simulink model "EQM"  (Simulink 7.8)
settings: Solver=FixedStepDiscrete  SolverMode=SingleTasking  StartTime=0.0  StopTime=t_end  FixedStep=dt_control  RelTol=1e-3
values from neighbouring files (symbols this model uses):
  dt_sim = 0.005    [Init.m]
  J = diag([0.25*m*(D/2)^2 0.25*m*(D/2)^2 0.5*m*(D/2)^2])    [Init.m]
  m = 1    [Init.m]
libraries: simulink x1
settings Model: Creator=ft14sl  LastModifiedBy=ft14sl
settings DataIOCC: LimitDataPoints=off  SaveOutput=off  SignalLogging=off  DSMLogging=off  SaveTime=off
settings DebuggingCC: ConsistencyChecking=error  SignalInfNanChecking=error  SignalRangeChecking=error  AlgebraicLoopMsg=error  ArtificialAlgebraicLoopMsg=error  SaveWithDisabledLinksMsg=error  SaveWithParameterizedLinksMsg=error  UnderspecifiedInitializationDetection=Simplified  MergeDetectMultiDrivingBlocksExec=error  BlockPriorityViolationMsg=error  MinStepSizeMsg=error  TimeAdjustmentMsg=warning  SolverPrmCheckMsg=error  InheritedTsInSrcMsg=error  DiscreteInheritContinuousMsg=error  SingleTaskRateTransMsg=error  TasksWithSamePriorityMsg=error  SigSpecEnsureSampleTimeMsg=error  CheckMatrixSingularityMsg=error  IntegerOverflowMsg=error  ParameterUnderflowMsg=error  ParameterPrecisionLossMsg=error  ParameterTunabilityLossMsg=error  FixptConstUnderflowMsg=error  FixptConstOverflowMsg=error  FixptConstPrecisionLossMsg=error  UnderSpecifiedDataTypeMsg=error  UnnecessaryDatatypeConvMsg=warning  VectorMatrixConversionMsg=error  SignalLabelMismatchMsg=error  UnconnectedInputMsg=error  UnconnectedOutputMsg=error  UnconnectedLineMsg=error  SFcnCompatibilityMsg=error  UniqueDataStoreMsg=error  BusObjectLabelMismatch=error  RootOutportRequireBusObject=error  ModelReferenceIOMsg=error  ModelReferenceVersionMismatchMessage=error  ModelReferenceIOMismatchMessage=error  ModelReferenceCSMismatchMessage=error  UnknownTsInhSupMsg=error  ModelReferenceDataLoggingMessage=error  SimStateInterfaceChecksumMismatchMsg=error  StrictBusMsg=ErrorOnBusTreatedAsVector  NonBusSignalsTreatedAsBus=error  SFUnusedDataAndEventsDiag=error  SFUnexpectedBacktrackingDiag=error  SFInvalidInputDataAccessInChartInitDiag=error  SFNoUnconditionalDefaultTransitionDiag=error  SFTransitionOutsideNaturalParentDiag=error  SFUnconditionalTransitionShadowingDiag=error

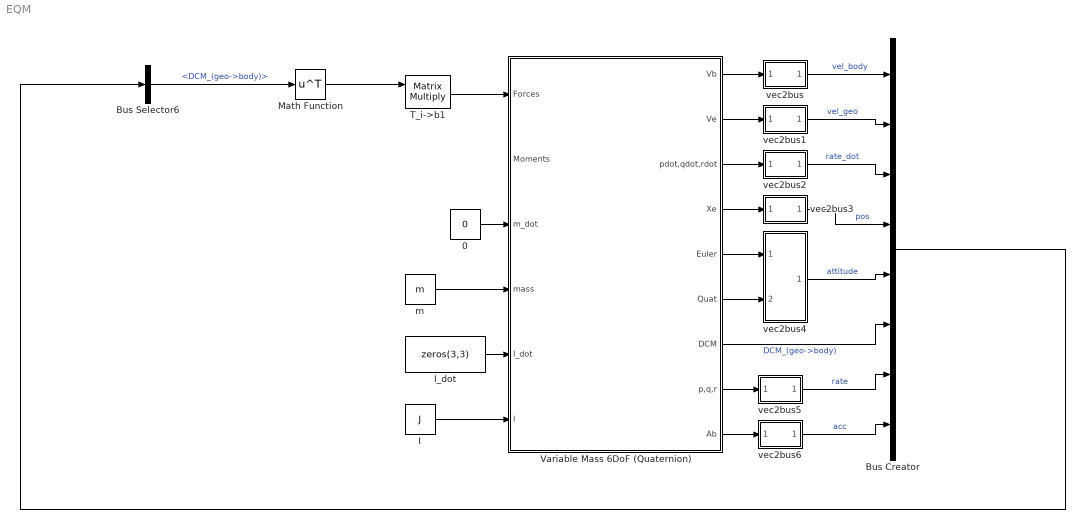
== system EQM ==
  0 : Constant  Value=0
  Bus Creator : BusCreator  Inputs=8
  Bus Selector6 : BusSelector  OutputSignals=DCM_(geo->body)
  I : Constant  Value=J
  I_dot : Constant  Value=zeros(3,3)
  Math Function : Math  Operator=transpose  SaturateOnIntegerOverflow=on
  T_i->b1 : Product  Multiplication=Matrix(*)  SaturateOnIntegerOverflow=on  OutDataTypeStr=Inherit: Same as first input
  Variable Mass 6DoF (Quaternion) : Subsystem  mask{xme_0=[0 0 0], Vm_0=[0 0 0], eul_0=[0 0 0], pm_0=[0 0 0], dt_sim=dt_sim}
      mask prompts: xme_0 "Inertial position in inertial axes [Xe, Ye Ze]"; Vm_0 "Inertial velocity in body axes [u, v, w]"; eul_0 "Inertial Euler orientation [roll, pitch, yaw]"; pm_0 "Inertial body rotation rates[p, q, r]"; dt_sim "Sample Time for quaternion integration"
      mask help:
      | Variable Mass 6DoF (Quaternion)
      | (rebuild from MATLAB AeroSpace Blockset)
      mask Help:
      | Inputs and Outputs
      | 
      | The first input to the block is a vector containing the three applied forces.
      | The second input is a vector containing the three applied moments.
      | The third input is a scalar containing the rate of change of mass.
      | The fourth input is a scalar containing the mass
      | The fifth input is a 3-by-3 matrix for the rate of change of inertia tensor matrix.
      | The sixth input is a 3-by-3 matrix for the inertia tensor matrix.
      | 
      | The first output is a three-element vector containing the velocity in the Earth-fixed reference frame.
      | The second output is a three-element vector containing the position in the Earth-fixed reference frame.
      | The third output is a three-element vector containing the Euler rotation angles [roll, pitch, yaw], in radians.
      | The fourth output is a 3-by-3 matrix for the coordinate transformation from Earth-fixed axes to body-fixed axes.
      | The fifth output is a three-element vector containing the velocity in the body-fixed frame.
      | The sixth output is a three-element vector containing the angular rates in body-fixed axes, in radians per second.
      | The seventh output is a three-element vector containing the angular accelerations in body-fixed axes, in radians per second. The eighth output is a three-element vector containing the accelerations in body-fixed axes.
      mask Display:
      | port_label('input',1,'F_xyz (N)')
      | port_label('input',2,'M_xyz (Nm)')
      | port_label('input',3,'dm/dt (kg/s)')
      | port_label('input',4,'m (kg)')
      | port_label('input',5,'dI/dt (kgm^2/s)')
      | port_label('input',6,'I (kgm^2)')
      | port_label('output',1,'Vb (m/s)')
      | port_label('output',2,'Ve (m/s)')
      | port_label('output',3,'pqrdot')
      | port_label('output',4,'Xe')
      | port_label('output',5,'phi theta psi (rad)')
      | port_label('output',6,'quaternions')
      | port_label('output',7,'DCM')
      | port_label('output',8,'pqr')
      | port_label('output',9,'Ab (m/s^2)')
  m : Constant  Value=m
  vec2bus : Subsystem
  vec2bus1 : Subsystem
  vec2bus2 : Subsystem
  vec2bus3 : Subsystem
  vec2bus4 : Subsystem
  vec2bus5 : Subsystem
  vec2bus6 : Subsystem
  wires:
  T_i->b1/1 -> Variable Mass 6DoF (Quaternion)/1(Forces)
  vec2bus6/1(bus) -> Bus Creator/8  "acc"
  vec2bus5/1(bus) -> Bus Creator/7  "rate"
  Variable Mass 6DoF (Quaternion)/7(DCM) -> Bus Creator/6  "DCM_(geo->body)"
  vec2bus4/1(bus) -> Bus Creator/5  "attitude"
  vec2bus3/1(bus) -> Bus Creator/4  "pos"
  vec2bus2/1(bus) -> Bus Creator/3  "rate_dot"
  vec2bus1/1(bus) -> Bus Creator/2  "vel_geo"
  vec2bus/1(bus) -> Bus Creator/1  "vel_body"
  Variable Mass 6DoF (Quaternion)/6(Quat) -> vec2bus4/2(quat)
  Variable Mass 6DoF (Quaternion)/9(Ab) -> vec2bus6/1(vec)
  Variable Mass 6DoF (Quaternion)/8(p,q,r) -> vec2bus5/1(vec)
  Variable Mass 6DoF (Quaternion)/5(Euler) -> vec2bus4/1(euler)
  Variable Mass 6DoF (Quaternion)/4(Xe) -> vec2bus3/1(vec)
  Variable Mass 6DoF (Quaternion)/3(pdot,qdot,rdot) -> vec2bus2/1(vec)
  Variable Mass 6DoF (Quaternion)/2(Ve) -> vec2bus1/1(vec)
  Variable Mass 6DoF (Quaternion)/1(Vb) -> vec2bus/1(vec)
  I/1 -> Variable Mass 6DoF (Quaternion)/6(I)
  I_dot/1 -> Variable Mass 6DoF (Quaternion)/5(I_dot)
  m/1 -> Variable Mass 6DoF (Quaternion)/4(mass)
  0/1 -> Variable Mass 6DoF (Quaternion)/3(m_dot)
  Math Function/1 -> T_i->b1/1
  Bus Selector6/1 -> Math Function/1  "<DCM_(geo->body)>"
  Bus Creator/1 -> Bus Selector6/1

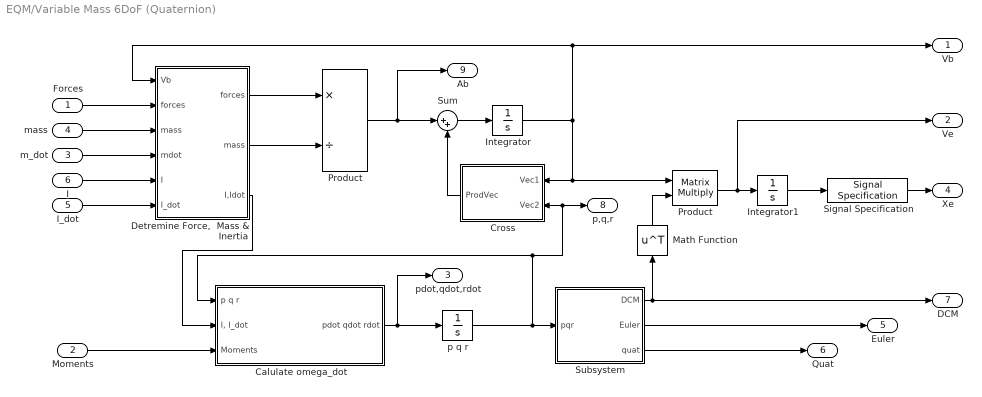
== system EQM/Variable Mass 6DoF (Quaternion) ==
  Forces : Inport
  Moments : Inport  Port=2
  m_dot : Inport  Port=3
  mass : Inport  Port=4
  I_dot : Inport  Port=5
  I : Inport  Port=6
  Calulate omega_dot : Subsystem
  Cross : Subsystem
  "Detremine Force,  Mass & Inertia" : Subsystem
  Integrator : Integrator  InitialCondition=Vm_0
  Integrator1 : Integrator  InitialCondition=xme_0
  Math Function : Math  Operator=transpose  SaturateOnIntegerOverflow=on
  Product : Product  Inputs=*/  SaturateOnIntegerOverflow=on  OutDataTypeStr=Inherit: Same as first input
  "Product " : Product  Multiplication=Matrix(*)  SaturateOnIntegerOverflow=on  OutDataTypeStr=Inherit: Same as first input
  Signal Specification : SignalSpecification  OutDataTypeStr=double
  Subsystem : Subsystem
  Sum : Sum  Inputs=|++  SaturateOnIntegerOverflow=on
  p q r : Integrator
  Vb : Outport
  Ve : Outport  Port=2
  pdot,qdot,rdot : Outport  Port=3
  Xe : Outport  Port=4
  Euler : Outport  Port=5
  Quat : Outport  Port=6
  DCM : Outport  Port=7
  p,q,r : Outport  Port=8
  Ab : Outport  Port=9
  wires:
  Subsystem/2(Euler) -> Euler/1
  Integrator1/1 -> Signal Specification/1
  "Product "/1 -> Ve/1, Integrator1/1
  "Detremine Force,  Mass & Inertia"/3(I,Idot) -> Calulate omega_dot/2("I, I_dot")
  Moments/1 -> Calulate omega_dot/3(Moments)
  Calulate omega_dot/1(pdot qdot rdot) -> pdot,qdot,rdot/1, p q r/1
  p q r/1 -> Calulate omega_dot/1(p q r), Cross/2(Vec2), p,q,r/1, Subsystem/1(pqr)
  Subsystem/1(DCM) -> DCM/1, Math Function/1
  Math Function/1 -> "Product "/2
  Cross/1(ProdVec) -> Sum/2
  Sum/1 -> Integrator/1
  Integrator/1 -> Vb/1, "Detremine Force,  Mass & Inertia"/1(Vb), "Product "/1, Cross/1(Vec1)
  Product/1 -> Sum/1, Ab/1
  "Detremine Force,  Mass & Inertia"/2("mass ") -> Product/2
  "Detremine Force,  Mass & Inertia"/1("forces ") -> Product/1
  I_dot/1 -> "Detremine Force,  Mass & Inertia"/6(I_dot)
  I/1 -> "Detremine Force,  Mass & Inertia"/5(I)
  m_dot/1 -> "Detremine Force,  Mass & Inertia"/4(mdot)
  mass/1 -> "Detremine Force,  Mass & Inertia"/3(mass)
  Forces/1 -> "Detremine Force,  Mass & Inertia"/2(forces)
  Subsystem/3(quat) -> Quat/1
  Signal Specification/1 -> Xe/1

== system EQM/vec2bus ==
  vec : Inport
  Bus Creator : BusCreator  Inputs=3
  Demux : Demux  Outputs=3
  bus : Outport
  wires:
  Demux/1 -> Bus Creator/1  "ub"
  Demux/2 -> Bus Creator/2  "vb"
  Demux/3 -> Bus Creator/3  "wb"
  Bus Creator/1 -> bus/1
  vec/1 -> Demux/1

== system EQM/vec2bus1 ==
  vec : Inport
  Bus Creator : BusCreator  Inputs=3
  Demux : Demux  Outputs=3
  bus : Outport
  wires:
  vec/1 -> Demux/1
  Bus Creator/1 -> bus/1
  Demux/3 -> Bus Creator/3  "wg"
  Demux/2 -> Bus Creator/2  "vg"
  Demux/1 -> Bus Creator/1  "ug"

== system EQM/vec2bus2 ==
  vec : Inport
  Bus Creator : BusCreator  Inputs=3
  Demux : Demux  Outputs=3
  bus : Outport
  wires:
  Demux/1 -> Bus Creator/1  "pdot"
  Demux/2 -> Bus Creator/2  "qdot"
  Demux/3 -> Bus Creator/3  "rdot"
  Bus Creator/1 -> bus/1
  vec/1 -> Demux/1

== system EQM/vec2bus3 ==
  vec : Inport
  Bus Creator : BusCreator  Inputs=3
  Demux : Demux  Outputs=3
  bus : Outport
  wires:
  vec/1 -> Demux/1
  Bus Creator/1 -> bus/1
  Demux/3 -> Bus Creator/3  "z"
  Demux/2 -> Bus Creator/2  "y"
  Demux/1 -> Bus Creator/1  "x"

== system EQM/vec2bus4 ==
  euler : Inport
  quat : Inport  Port=2
  Bus Creator : BusCreator  Inputs=7
  Demux : Demux  Outputs=3
  Demux1 : Demux
  bus : Outport
  wires:
  Demux/1 -> Bus Creator/1  "phi"
  Demux/2 -> Bus Creator/2  "theta"
  Demux/3 -> Bus Creator/3  "psi"
  Demux1/1 -> Bus Creator/4
  Demux1/2 -> Bus Creator/5
  Demux1/3 -> Bus Creator/6
  Demux1/4 -> Bus Creator/7
  euler/1 -> Demux/1
  Bus Creator/1 -> bus/1
  quat/1 -> Demux1/1

== system EQM/vec2bus5 ==
  vec : Inport
  Bus Creator : BusCreator  Inputs=3
  Demux : Demux  Outputs=3
  bus : Outport
  wires:
  vec/1 -> Demux/1
  Bus Creator/1 -> bus/1
  Demux/3 -> Bus Creator/3  "r"
  Demux/2 -> Bus Creator/2  "q"
  Demux/1 -> Bus Creator/1  "p"

== system EQM/vec2bus6 ==
  vec : Inport
  Bus Creator : BusCreator  Inputs=3
  Demux : Demux  Outputs=3
  bus : Outport
  wires:
  Demux/1 -> Bus Creator/1  "ax"
  Demux/2 -> Bus Creator/2  "ay"
  Demux/3 -> Bus Creator/3  "az"
  Bus Creator/1 -> bus/1
  vec/1 -> Demux/1

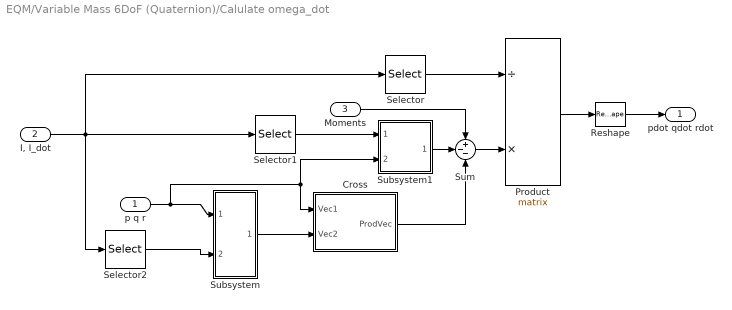
== system EQM/Variable Mass 6DoF (Quaternion)/Calulate omega_dot ==
  p q r : Inport
  "I, I_dot" : Inport  Port=2
  Moments : Inport  Port=3
  Cross : Subsystem
  Product : Product  Inputs=/*  Multiplication=Matrix(*)  SaturateOnIntegerOverflow=on  OutDataTypeStr=Inherit: Same as first input
  Reshape : Reshape
  Selector : Selector  NumberOfDimensions=2  InputPortWidth=3  IndexOptions=Index vector (dialog),Select all  Indices=1:3,-1  OutputSizes=1
  Selector1 : Selector  NumberOfDimensions=2  InputPortWidth=3  IndexOptions=Index vector (dialog),Select all  Indices=4:6,-1  OutputSizes=1
  Selector2 : Selector  NumberOfDimensions=2  InputPortWidth=3  IndexOptions=Index vector (dialog),Select all  Indices=1:3,-1  OutputSizes=1
  Subsystem : Subsystem
  Subsystem1 : Subsystem
  Sum : Sum  Inputs=+--  SaturateOnIntegerOverflow=on
  pdot qdot rdot : Outport
  wires:
  Cross/1(ProdVec) -> Sum/3
  Product/1 -> Reshape/1
  Subsystem/1(I*w) -> Cross/2(Vec2)
  Selector2/1 -> Subsystem/2(Inertia)
  p q r/1 -> Subsystem1/2(p q r), Cross/1(Vec1), Subsystem/1(p q r)
  Moments/1 -> Sum/1
  Reshape/1 -> pdot qdot rdot/1
  Sum/1 -> Product/2
  Subsystem1/1(Id*w) -> Sum/2
  Selector1/1 -> Subsystem1/1(I_dot)
  Selector/1 -> Product/1
  "I, I_dot"/1 -> Selector2/1, Selector1/1, Selector/1

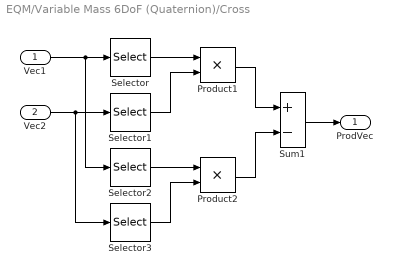
== system EQM/Variable Mass 6DoF (Quaternion)/Cross ==
  Vec1 : Inport
  Vec2 : Inport  Port=2
  Product1 : Product  SaturateOnIntegerOverflow=on  InputSameDT=on  OutDataTypeStr=Inherit: Same as first input
  Product2 : Product  SaturateOnIntegerOverflow=on  InputSameDT=on  OutDataTypeStr=Inherit: Same as first input
  Selector : Selector  InputPortWidth=3  IndexOptions=Index vector (dialog)  Indices=[2 3 1]  OutputSizes=1
  Selector1 : Selector  InputPortWidth=3  IndexOptions=Index vector (dialog)  Indices=[3 1 2]  OutputSizes=1
  Selector2 : Selector  InputPortWidth=3  IndexOptions=Index vector (dialog)  Indices=[3 1 2]  OutputSizes=1
  Selector3 : Selector  InputPortWidth=3  IndexOptions=Index vector (dialog)  Indices=[2 3 1]  OutputSizes=1
  Sum1 : Sum  Inputs=+-  SaturateOnIntegerOverflow=on  InputSameDT=on  OutDataTypeStr=Inherit: Same as first input
  ProdVec : Outport
  wires:
  Sum1/1 -> ProdVec/1
  Product2/1 -> Sum1/2
  Product1/1 -> Sum1/1
  Selector3/1 -> Product2/2
  Selector2/1 -> Product2/1
  Selector1/1 -> Product1/2
  Selector/1 -> Product1/1
  Vec2/1 -> Selector1/1, Selector3/1
  Vec1/1 -> Selector/1, Selector2/1

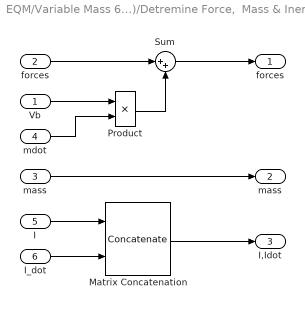
== system EQM/Variable Mass 6DoF (Quaternion)/Detremine Force,  Mass & Inertia ==
  Vb : Inport
  forces : Inport  Port=2
  mass : Inport  Port=3
  mdot : Inport  Port=4
  I : Inport  Port=5
  I_dot : Inport  Port=6
  Matrix Concatenation : Concatenate  Mode=Multidimensional array
  Product : Product  SaturateOnIntegerOverflow=on  OutDataTypeStr=Inherit: Same as first input
  Sum : Sum  Inputs=|++  SaturateOnIntegerOverflow=on
  "forces " : Outport
  "mass " : Outport  Port=2
  I,Idot : Outport  Port=3
  wires:
  Matrix Concatenation/1 -> I,Idot/1
  mass/1 -> "mass "/1
  Sum/1 -> "forces "/1
  forces/1 -> Sum/1
  Vb/1 -> Product/1
  mdot/1 -> Product/2
  I_dot/1 -> Matrix Concatenation/2
  I/1 -> Matrix Concatenation/1
  Product/1 -> Sum/2

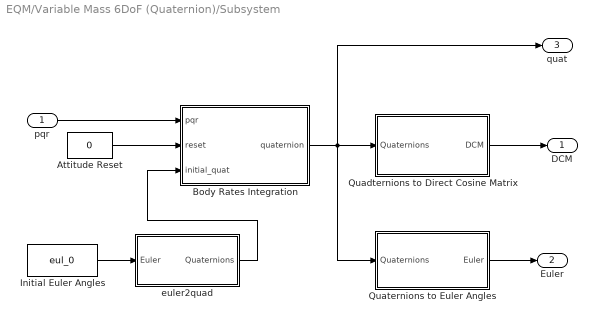
== system EQM/Variable Mass 6DoF (Quaternion)/Subsystem ==
  pqr : Inport
  Attitude Reset : Constant  Value=0
  Body Rates Integration : Subsystem  mask{dt_sim=dt_sim}
      mask prompts: dt_sim "Sample Time"
  Initial Euler Angles : Constant  Value=eul_0
  Quadternions to Direct Cosine Matrix : Subsystem
  "Quaternions to Euler Angles " : Subsystem
  euler2quad : Subsystem
  DCM : Outport
  Euler : Outport  Port=2
  quat : Outport  Port=3
  wires:
  "Quaternions to Euler Angles "/1(Euler) -> Euler/1
  Quadternions to Direct Cosine Matrix/1(DCM) -> DCM/1
  Body Rates Integration/1(quaternion) -> Quadternions to Direct Cosine Matrix/1(Quaternions), quat/1, "Quaternions to Euler Angles "/1(Quaternions)
  Initial Euler Angles/1 -> euler2quad/1(Euler)
  pqr/1 -> Body Rates Integration/1(pqr)
  euler2quad/1(Quaternions) -> Body Rates Integration/3(initial_quat)
  Attitude Reset/1 -> Body Rates Integration/2(reset)

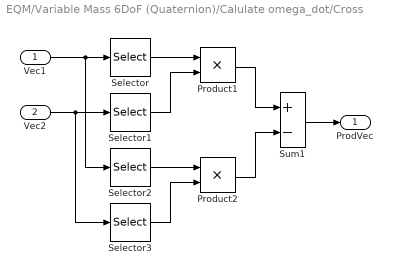
== system EQM/Variable Mass 6DoF (Quaternion)/Calulate omega_dot/Cross ==
  Vec1 : Inport
  Vec2 : Inport  Port=2
  Product1 : Product  SaturateOnIntegerOverflow=on  InputSameDT=on  OutDataTypeStr=Inherit: Same as first input
  Product2 : Product  SaturateOnIntegerOverflow=on  InputSameDT=on  OutDataTypeStr=Inherit: Same as first input
  Selector : Selector  InputPortWidth=3  IndexOptions=Index vector (dialog)  Indices=[2 3 1]  OutputSizes=1
  Selector1 : Selector  InputPortWidth=3  IndexOptions=Index vector (dialog)  Indices=[3 1 2]  OutputSizes=1
  Selector2 : Selector  InputPortWidth=3  IndexOptions=Index vector (dialog)  Indices=[3 1 2]  OutputSizes=1
  Selector3 : Selector  InputPortWidth=3  IndexOptions=Index vector (dialog)  Indices=[2 3 1]  OutputSizes=1
  Sum1 : Sum  Inputs=+-  SaturateOnIntegerOverflow=on  InputSameDT=on  OutDataTypeStr=Inherit: Same as first input
  ProdVec : Outport
  wires:
  Sum1/1 -> ProdVec/1
  Product2/1 -> Sum1/2
  Product1/1 -> Sum1/1
  Selector3/1 -> Product2/2
  Selector2/1 -> Product2/1
  Selector1/1 -> Product1/2
  Selector/1 -> Product1/1
  Vec2/1 -> Selector1/1, Selector3/1
  Vec1/1 -> Selector/1, Selector2/1

== system EQM/Variable Mass 6DoF (Quaternion)/Calulate omega_dot/Subsystem ==
  p q r : Inport
  Inertia : Inport  Port=2
  Product2 : Product  Multiplication=Matrix(*)  SaturateOnIntegerOverflow=on  OutDataTypeStr=Inherit: Same as first input
  I*w : Outport
  wires:
  p q r/1 -> Product2/2
  Inertia/1 -> Product2/1
  Product2/1 -> I*w/1

== system EQM/Variable Mass 6DoF (Quaternion)/Calulate omega_dot/Subsystem1 ==
  I_dot : Inport
  p q r : Inport  Port=2
  Product2 : Product  Multiplication=Matrix(*)  SaturateOnIntegerOverflow=on  OutDataTypeStr=Inherit: Same as first input
  Id*w : Outport
  wires:
  I_dot/1 -> Product2/1
  Product2/1 -> Id*w/1
  p q r/1 -> Product2/2

== system EQM/Variable Mass 6DoF (Quaternion)/Subsystem/Body Rates Integration ==
  pqr : Inport
  reset : Inport  Port=2
  initial_quat : Inport  Port=3
  Rate Integration : Subsystem  mask{dt_sim=dt_sim}
      mask prompts: dt_sim "Sample Time"
  Unit Delay Resettable External IC : simulink/Additional Math & Discrete/Additional Discrete/Unit Delay Resettable External IC  tsamp=dt_sim
  quaternion : Outport
  wires:
  initial_quat/1 -> Unit Delay Resettable External IC/3
  pqr/1 -> Rate Integration/1(p q r)
  reset/1 -> Unit Delay Resettable External IC/2
  Unit Delay Resettable External IC/1 -> Rate Integration/2(q0 q1 q2 q3)
  Rate Integration/1(q_prod) -> quaternion/1, Unit Delay Resettable External IC/1  "quat"

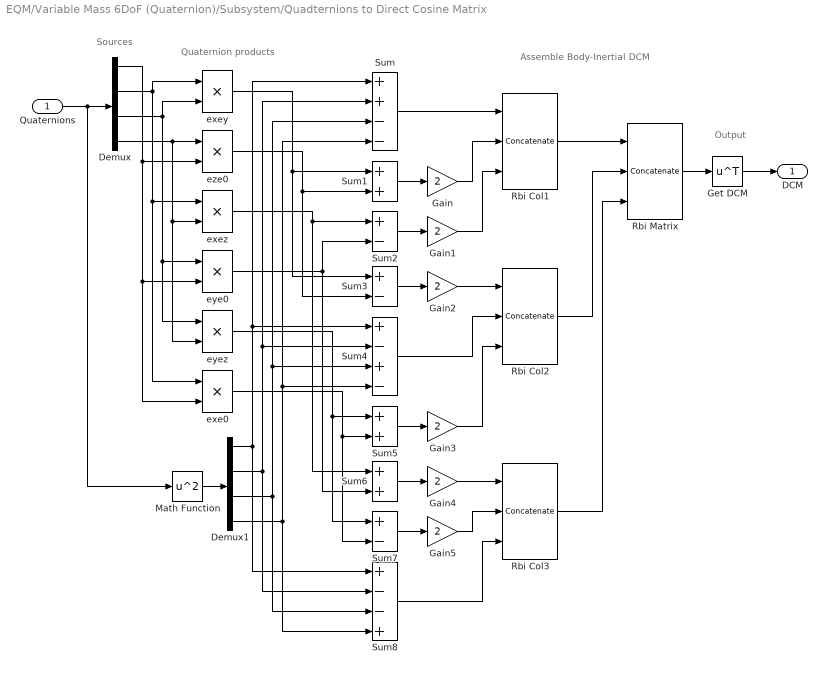
== system EQM/Variable Mass 6DoF (Quaternion)/Subsystem/Quadternions to Direct Cosine Matrix ==
  note: Output
  note: Quaternion products
  note: Assemble Body-Inertial DCM
  note: Sources
  Quaternions : Inport  PortDimensions=[4 1]
  Demux : Demux
  Demux1 : Demux
  Gain{,1..5} (6 alike) : Gain  Gain=2  SaturateOnIntegerOverflow=on  OutDataTypeStr=Inherit: Same as input  ParamDataTypeStr=Inherit: Same as input
  Get DCM : Math  Operator=transpose  SaturateOnIntegerOverflow=on
  Math Function : Math  Operator=square  SaturateOnIntegerOverflow=on
  Rbi Matrix : Concatenate  NumInputs=3  Mode=Multidimensional array  ConcatenateDimension=2
  Rbi Col1 : Concatenate  NumInputs=3  Mode=Multidimensional array
  Rbi Col2 : Concatenate  NumInputs=3  Mode=Multidimensional array
  Rbi Col3 : Concatenate  NumInputs=3  Mode=Multidimensional array
  Sum : Sum  Inputs=++--  SaturateOnIntegerOverflow=on  InputSameDT=on  OutDataTypeStr=Inherit: Same as first input
  Sum1 : Sum  SaturateOnIntegerOverflow=on  InputSameDT=on  OutDataTypeStr=Inherit: Same as first input
  Sum2 : Sum  Inputs=+-  SaturateOnIntegerOverflow=on  InputSameDT=on  OutDataTypeStr=Inherit: Same as first input
  Sum3 : Sum  Inputs=+-  SaturateOnIntegerOverflow=on  InputSameDT=on  OutDataTypeStr=Inherit: Same as first input
  Sum4 : Sum  Inputs=+-+-  SaturateOnIntegerOverflow=on  InputSameDT=on  OutDataTypeStr=Inherit: Same as first input
  Sum5 : Sum  SaturateOnIntegerOverflow=on  InputSameDT=on  OutDataTypeStr=Inherit: Same as first input
  Sum6 : Sum  SaturateOnIntegerOverflow=on  InputSameDT=on  OutDataTypeStr=Inherit: Same as first input
  Sum7 : Sum  Inputs=+-  SaturateOnIntegerOverflow=on  InputSameDT=on  OutDataTypeStr=Inherit: Same as first input
  Sum8 : Sum  Inputs=+--+  SaturateOnIntegerOverflow=on  InputSameDT=on  OutDataTypeStr=Inherit: Same as first input
  exe0 : Product  SaturateOnIntegerOverflow=on  InputSameDT=on  OutDataTypeStr=Inherit: Same as first input
  exey : Product  SaturateOnIntegerOverflow=on  InputSameDT=on  OutDataTypeStr=Inherit: Same as first input
  exez : Product  SaturateOnIntegerOverflow=on  InputSameDT=on  OutDataTypeStr=Inherit: Same as first input
  eye0 : Product  SaturateOnIntegerOverflow=on  InputSameDT=on  OutDataTypeStr=Inherit: Same as first input
  eyez : Product  SaturateOnIntegerOverflow=on  InputSameDT=on  OutDataTypeStr=Inherit: Same as first input
  eze0 : Product  SaturateOnIntegerOverflow=on  InputSameDT=on  OutDataTypeStr=Inherit: Same as first input
  DCM : Outport
  wires:
  Get DCM/1 -> DCM/1
  Rbi Matrix/1 -> Get DCM/1
  Sum8/1 -> Rbi Col3/3
  Gain5/1 -> Rbi Col3/2
  Gain4/1 -> Rbi Col3/1
  Rbi Col3/1 -> Rbi Matrix/3
  Sum7/1 -> Gain5/1
  Sum6/1 -> Gain4/1
  Rbi Col2/1 -> Rbi Matrix/2
  Gain3/1 -> Rbi Col2/3
  Sum4/1 -> Rbi Col2/2
  Gain2/1 -> Rbi Col2/1
  Sum5/1 -> Gain3/1
  Sum3/1 -> Gain2/1
  Rbi Col1/1 -> Rbi Matrix/1
  Gain1/1 -> Rbi Col1/3
  Gain/1 -> Rbi Col1/2
  Sum/1 -> Rbi Col1/1
  Sum2/1 -> Gain1/1
  Sum1/1 -> Gain/1
  exe0/1 -> Sum5/2, Sum7/2
  eyez/1 -> Sum5/1, Sum7/1
  eye0/1 -> Sum2/2, Sum6/2
  exez/1 -> Sum2/1, Sum6/1
  eze0/1 -> Sum1/2, Sum3/2
  exey/1 -> Sum1/1, Sum3/1
  Math Function/1 -> Demux1/1
  Demux/4 -> eze0/1, exez/2, eyez/2
  Demux/3 -> exey/2, eye0/1, eyez/1
  Demux/2 -> exey/1, exez/1, exe0/1
  Demux/1 -> eze0/2, eye0/2, exe0/2
  Quaternions/1 -> Demux/1, Math Function/1
  Demux1/1 -> Sum/1, Sum4/1, Sum8/1
  Demux1/2 -> Sum/2, Sum4/2, Sum8/2
  Demux1/3 -> Sum/3, Sum4/3, Sum8/3
  Demux1/4 -> Sum/4, Sum4/4, Sum8/4

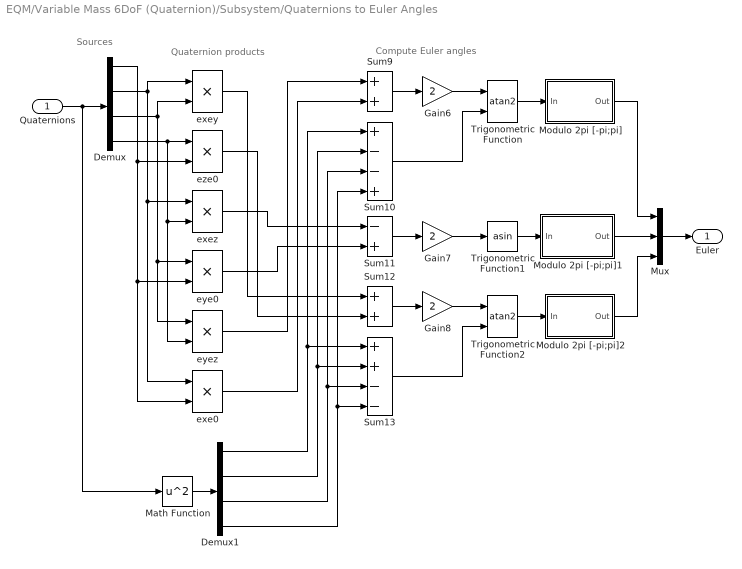
== system EQM/Variable Mass 6DoF (Quaternion)/Subsystem/Quaternions to Euler Angles  ==
  note: Compute Euler angles
  note: Sources
  note: Quaternion products
  Quaternions : Inport  PortDimensions=[4 1]
  Demux : Demux
  Demux1 : Demux
  Gain6 : Gain  Gain=2  SaturateOnIntegerOverflow=on  OutDataTypeStr=Inherit: Same as input  ParamDataTypeStr=Inherit: Same as input
  Gain7 : Gain  Gain=2  SaturateOnIntegerOverflow=on  OutDataTypeStr=Inherit: Same as input  ParamDataTypeStr=Inherit: Same as input
  Gain8 : Gain  Gain=2  SaturateOnIntegerOverflow=on  OutDataTypeStr=Inherit: Same as input  ParamDataTypeStr=Inherit: Same as input
  Math Function : Math  Operator=square  SaturateOnIntegerOverflow=on
  Modulo 2pi [-pi;pi] : Subsystem
  Modulo 2pi [-pi;pi]1 : Subsystem
  Modulo 2pi [-pi;pi]2 : Subsystem
  Mux : Mux  Inputs=3
  Sum10 : Sum  Inputs=+--+  SaturateOnIntegerOverflow=on  InputSameDT=on  OutDataTypeStr=Inherit: Same as first input
  Sum11 : Sum  Inputs=-+  SaturateOnIntegerOverflow=on  InputSameDT=on  OutDataTypeStr=Inherit: Same as first input
  Sum12 : Sum  SaturateOnIntegerOverflow=on  InputSameDT=on  OutDataTypeStr=Inherit: Same as first input
  Sum13 : Sum  Inputs=++--  SaturateOnIntegerOverflow=on  InputSameDT=on  OutDataTypeStr=Inherit: Same as first input
  Sum9 : Sum  SaturateOnIntegerOverflow=on  InputSameDT=on  OutDataTypeStr=Inherit: Same as first input
  Trigonometric Function : Trigonometry  Operator=atan2
  Trigonometric Function1 : Trigonometry  Operator=asin
  Trigonometric Function2 : Trigonometry  Operator=atan2
  exe0 : Product  SaturateOnIntegerOverflow=on  InputSameDT=on  OutDataTypeStr=Inherit: Same as first input
  exey : Product  SaturateOnIntegerOverflow=on  InputSameDT=on  OutDataTypeStr=Inherit: Same as first input
  exez : Product  SaturateOnIntegerOverflow=on  InputSameDT=on  OutDataTypeStr=Inherit: Same as first input
  eye0 : Product  SaturateOnIntegerOverflow=on  InputSameDT=on  OutDataTypeStr=Inherit: Same as first input
  eyez : Product  SaturateOnIntegerOverflow=on  InputSameDT=on  OutDataTypeStr=Inherit: Same as first input
  eze0 : Product  SaturateOnIntegerOverflow=on  InputSameDT=on  OutDataTypeStr=Inherit: Same as first input
  Euler : Outport
  wires:
  Sum9/1 -> Gain6/1
  Gain6/1 -> Trigonometric Function/1
  Sum10/1 -> Trigonometric Function/2
  Sum11/1 -> Gain7/1
  Gain7/1 -> Trigonometric Function1/1
  Sum12/1 -> Gain8/1
  Gain8/1 -> Trigonometric Function2/1
  Sum13/1 -> Trigonometric Function2/2
  Trigonometric Function1/1 -> Modulo 2pi [-pi;pi]1/1(In)
  Trigonometric Function/1 -> Modulo 2pi [-pi;pi]/1(In)
  Trigonometric Function2/1 -> Modulo 2pi [-pi;pi]2/1(In)
  Quaternions/1 -> Demux/1, Math Function/1
  Demux/1 -> eze0/2, eye0/2, exe0/2
  Demux/2 -> exey/1, exez/1, exe0/1
  Demux/3 -> exey/2, eye0/1, eyez/1
  Demux/4 -> eze0/1, exez/2, eyez/2
  Demux1/1 -> Sum10/1, Sum13/1
  Demux1/2 -> Sum10/2, Sum13/2
  Demux1/3 -> Sum10/3, Sum13/3
  Demux1/4 -> Sum10/4, Sum13/4
  Math Function/1 -> Demux1/1
  exey/1 -> Sum12/1
  eze0/1 -> Sum12/2
  exez/1 -> Sum11/1
  eye0/1 -> Sum11/2
  eyez/1 -> Sum9/1
  exe0/1 -> Sum9/2
  Mux/1 -> Euler/1
  Modulo 2pi [-pi;pi]/1(Out) -> Mux/1
  Modulo 2pi [-pi;pi]1/1(Out) -> Mux/2
  Modulo 2pi [-pi;pi]2/1(Out) -> Mux/3

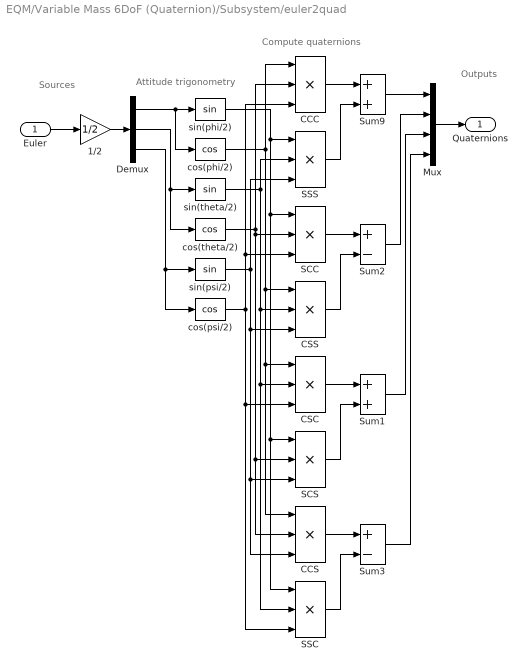
== system EQM/Variable Mass 6DoF (Quaternion)/Subsystem/euler2quad ==
  note: Sources
  note: Attitude trigonometry
  note: Compute quaternions
  note: Outputs
  Euler : Inport  PortDimensions=[3 1]
  1/2 : Gain  Gain=1/2  SaturateOnIntegerOverflow=on  OutDataTypeStr=Inherit: Same as input  ParamDataTypeStr=Inherit: Same as input
  CCC : Product  Inputs=3  SaturateOnIntegerOverflow=on  InputSameDT=on  OutDataTypeStr=Inherit: Same as first input
  CCS : Product  Inputs=3  SaturateOnIntegerOverflow=on  InputSameDT=on  OutDataTypeStr=Inherit: Same as first input
  CSC : Product  Inputs=3  SaturateOnIntegerOverflow=on  InputSameDT=on  OutDataTypeStr=Inherit: Same as first input
  CSS : Product  Inputs=3  SaturateOnIntegerOverflow=on  InputSameDT=on  OutDataTypeStr=Inherit: Same as first input
  Demux : Demux  Outputs=3
  Mux : Mux
  SCC : Product  Inputs=3  SaturateOnIntegerOverflow=on  InputSameDT=on  OutDataTypeStr=Inherit: Same as first input
  SCS : Product  Inputs=3  SaturateOnIntegerOverflow=on  InputSameDT=on  OutDataTypeStr=Inherit: Same as first input
  SSC : Product  Inputs=3  SaturateOnIntegerOverflow=on  InputSameDT=on  OutDataTypeStr=Inherit: Same as first input
  SSS : Product  Inputs=3  SaturateOnIntegerOverflow=on  InputSameDT=on  OutDataTypeStr=Inherit: Same as first input
  Sum1 : Sum  SaturateOnIntegerOverflow=on  InputSameDT=on  OutDataTypeStr=Inherit: Same as first input
  Sum2 : Sum  Inputs=+-  SaturateOnIntegerOverflow=on  InputSameDT=on  OutDataTypeStr=Inherit: Same as first input
  Sum3 : Sum  Inputs=+-  SaturateOnIntegerOverflow=on  InputSameDT=on  OutDataTypeStr=Inherit: Same as first input
  Sum9 : Sum  SaturateOnIntegerOverflow=on  InputSameDT=on  OutDataTypeStr=Inherit: Same as first input
  cos(phi/2) : Trigonometry  Operator=cos
  cos(psi/2) : Trigonometry  Operator=cos
  cos(theta/2) : Trigonometry  Operator=cos
  sin(phi/2) : Trigonometry
  sin(psi/2) : Trigonometry
  sin(theta/2) : Trigonometry
  Quaternions : Outport
  wires:
  Mux/1 -> Quaternions/1
  Euler/1 -> 1/2/1
  1/2/1 -> Demux/1
  Demux/1 -> sin(phi/2)/1, cos(phi/2)/1
  Demux/2 -> cos(theta/2)/1, sin(theta/2)/1
  Demux/3 -> cos(psi/2)/1, sin(psi/2)/1
  cos(psi/2)/1 -> CCC/3, SCC/3, SSC/3, CSC/3
  sin(psi/2)/1 -> SSS/3, CSS/3, CCS/3, SCS/3
  cos(theta/2)/1 -> SCC/2, CCS/2, SCS/2, CCC/2
  sin(theta/2)/1 -> SSS/2, CSS/2, SSC/2, CSC/2
  cos(phi/2)/1 -> CSS/1, CCS/1, CSC/1, CCC/1
  sin(phi/2)/1 -> SCC/1, SSC/1, SCS/1, SSS/1
  CCC/1 -> Sum9/1
  SSS/1 -> Sum9/2
  CSC/1 -> Sum1/1
  SCS/1 -> Sum1/2
  SCC/1 -> Sum2/1
  CSS/1 -> Sum2/2
  CCS/1 -> Sum3/1
  SSC/1 -> Sum3/2
  Sum9/1 -> Mux/1
  Sum2/1 -> Mux/2
  Sum1/1 -> Mux/3
  Sum3/1 -> Mux/4

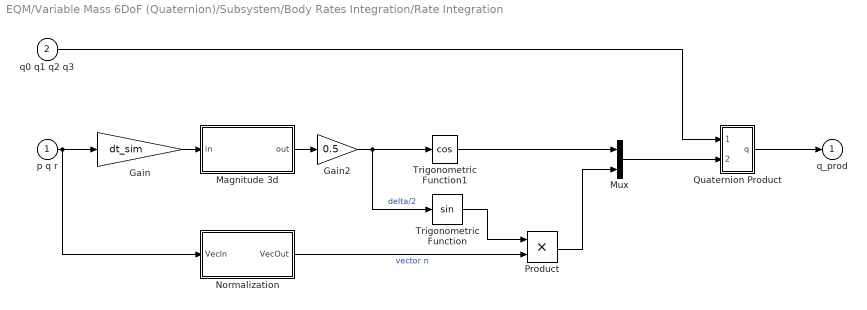
== system EQM/Variable Mass 6DoF (Quaternion)/Subsystem/Body Rates Integration/Rate Integration ==
  p q r : Inport
  q0 q1 q2 q3 : Inport  Port=2
  Gain : Gain  Gain=dt_sim
  Gain2 : Gain  Gain=0.5
  Magnitude 3d : Subsystem
      mask Type: Magnitude Square
      mask Description:
      | Magnitude of a 3-dimensional vector.
      | Input: 3-d vector (x,y,z).
      | Output: magn = sqrt(x^2 + y^2 + z^2).
      mask Help: Unmask block for more help.
      mask Display: disp('sqrt(x^2+y^2+z^2)')
  Mux : Mux  Inputs=2
  Normalization : Subsystem
      mask Type: Vector normalization
      mask Description: Normalize a vector, e = v/|v|.
      mask Help:
      | The block normalizes the input vector.
      | <P><B>Input:</B> the nx1 vector;</P>
      | <P><B>Output:</B> the nx1 unit vector.</P>
  Product : Product  RndMeth=Zero
  Quaternion Product : Subsystem
  Trigonometric Function : Trigonometry
  Trigonometric Function1 : Trigonometry  Operator=cos  OutputSignalType=real
  q_prod : Outport  InitialOutput=0
  wires:
  q0 q1 q2 q3/1 -> Quaternion Product/1(q_x)
  Quaternion Product/1(q) -> q_prod/1
  p q r/1 -> Gain/1, Normalization/1(VecIn)
  Magnitude 3d/1(out) -> Gain2/1
  Gain2/1 -> Trigonometric Function/1, Trigonometric Function1/1  "delta/2"
  Trigonometric Function1/1 -> Mux/1
  Trigonometric Function/1 -> Product/1
  Normalization/1(VecOut) -> Product/2  "vector n"
  Product/1 -> Mux/2
  Gain/1 -> Magnitude 3d/1(in)
  Mux/1 -> Quaternion Product/2(q_y)

== system EQM/Variable Mass 6DoF (Quaternion)/Subsystem/Quaternions to Euler Angles /Modulo 2pi [-pi;pi] ==
  In : Inport
  " " : Constant  Value=2*pi
  "  " : Constant  Value=pi
  "     " : Constant  Value=pi
  Math Function : Math  Operator=mod  SaturateOnIntegerOverflow=on
  Sum2 : Sum  Inputs=|++  SaturateOnIntegerOverflow=on  InputSameDT=on  OutDataTypeStr=Inherit: Same as first input
  Sum3 : Sum  Inputs=|+-  SaturateOnIntegerOverflow=on  InputSameDT=on  OutDataTypeStr=Inherit: Same as first input
  Out : Outport
  wires:
  In/1 -> Sum2/1
  Sum3/1 -> Out/1
  "     "/1 -> Sum2/2
  "  "/1 -> Sum3/2
  Sum2/1 -> Math Function/1
  Math Function/1 -> Sum3/1
  " "/1 -> Math Function/2

== system EQM/Variable Mass 6DoF (Quaternion)/Subsystem/Quaternions to Euler Angles /Modulo 2pi [-pi;pi]1 ==
  In : Inport
  " " : Constant  Value=2*pi
  "  " : Constant  Value=pi
  "     " : Constant  Value=pi
  Math Function : Math  Operator=mod  SaturateOnIntegerOverflow=on
  Sum2 : Sum  Inputs=|++  SaturateOnIntegerOverflow=on  InputSameDT=on  OutDataTypeStr=Inherit: Same as first input
  Sum3 : Sum  Inputs=|+-  SaturateOnIntegerOverflow=on  InputSameDT=on  OutDataTypeStr=Inherit: Same as first input
  Out : Outport
  wires:
  " "/1 -> Math Function/2
  Math Function/1 -> Sum3/1
  Sum2/1 -> Math Function/1
  "  "/1 -> Sum3/2
  "     "/1 -> Sum2/2
  Sum3/1 -> Out/1
  In/1 -> Sum2/1

== system EQM/Variable Mass 6DoF (Quaternion)/Subsystem/Quaternions to Euler Angles /Modulo 2pi [-pi;pi]2 ==
  In : Inport
  " " : Constant  Value=2*pi
  "  " : Constant  Value=pi
  "     " : Constant  Value=pi
  Math Function : Math  Operator=mod  SaturateOnIntegerOverflow=on
  Sum2 : Sum  Inputs=|++  SaturateOnIntegerOverflow=on  InputSameDT=on  OutDataTypeStr=Inherit: Same as first input
  Sum3 : Sum  Inputs=|+-  SaturateOnIntegerOverflow=on  InputSameDT=on  OutDataTypeStr=Inherit: Same as first input
  Out : Outport
  wires:
  In/1 -> Sum2/1
  Sum3/1 -> Out/1
  "     "/1 -> Sum2/2
  "  "/1 -> Sum3/2
  Sum2/1 -> Math Function/1
  Math Function/1 -> Sum3/1
  " "/1 -> Math Function/2

== system EQM/Variable Mass 6DoF (Quaternion)/Subsystem/Body Rates Integration/Rate Integration/Magnitude 3d ==
  note: magnitude for 3-d vector
  in : Inport
  Signal Specification : SignalSpecification  Dimensions=3
  magnitude square : Fcn  Expr=sqrt(u[1]*u[1]+u[2]*u[2]+u[3]*u[3])
  out : Outport
  wires:
  Signal Specification/1 -> magnitude square/1
  in/1 -> Signal Specification/1
  magnitude square/1 -> out/1

== system EQM/Variable Mass 6DoF (Quaternion)/Subsystem/Body Rates Integration/Rate Integration/Normalization ==
  VecIn : Inport
  Switch : Switch  Criteria=u2 > Threshold  Threshold=0.0001  InputSameDT=on
  Vector norm : Subsystem
      mask Type: Vector norm-2
      mask Description: Compute the 2-norm (magnitude) of a vector, |v| = sqrt(v'v)
  e/|e| : Product  Inputs=*/  SaturateOnIntegerOverflow=on  InputSameDT=on  OutDataTypeStr=Inherit: Same as first input
  VecOut : Outport
  wires:
  Vector norm/1(Mag) -> e/|e|/2, Switch/2
  e/|e|/1 -> Switch/1
  VecIn/1 -> e/|e|/1, Vector norm/1(Vec), Switch/3
  Switch/1 -> VecOut/1

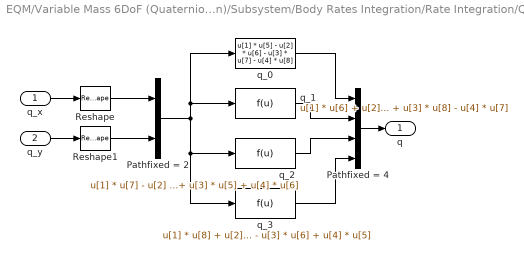
== system EQM/Variable Mass 6DoF (Quaternion)/Subsystem/Body Rates Integration/Rate Integration/Quaternion Product ==
  q_x : Inport
  q_y : Inport  Port=2
  Pathfixed = 2 : Mux  Inputs=2
  Pathfixed = 4 : Mux
  Reshape : Reshape
  Reshape1 : Reshape
  q_0 : Fcn  Expr=u[1] * u[5] - u[2] * u[6] - u[3] * u[7] - u[4] * u[8]
  q_1 : Fcn  Expr=u[1] * u[6] + u[2] * u[5] + u[3] * u[8] - u[4] * u[7]
  q_2 : Fcn  Expr=u[1] * u[7] - u[2] * u[8] + u[3] * u[5] + u[4] * u[6]
  q_3 : Fcn  Expr=u[1] * u[8] + u[2] * u[7] - u[3] * u[6] + u[4] * u[5]
  q : Outport
  wires:
  Reshape1/1 -> Pathfixed = 2/2
  Reshape/1 -> Pathfixed = 2/1
  Pathfixed = 2/1 -> q_0/1, q_1/1, q_2/1, q_3/1
  q_0/1 -> Pathfixed = 4/1
  q_1/1 -> Pathfixed = 4/2
  q_2/1 -> Pathfixed = 4/3
  q_3/1 -> Pathfixed = 4/4
  q_x/1 -> Reshape/1
  Pathfixed = 4/1 -> q/1
  q_y/1 -> Reshape1/1

== system EQM/Variable Mass 6DoF (Quaternion)/Subsystem/Body Rates Integration/Rate Integration/Normalization/Vector norm ==
  Vec : Inport
  Dot Product : DotProduct  InputSameDT=on  OutDataTypeStr=Inherit: Inherit via internal rule
  Sqrt : Sqrt  OutputSignalType=real  SaturateOnIntegerOverflow=on
  Mag : Outport
  wires:
  Sqrt/1 -> Mag/1
  Dot Product/1 -> Sqrt/1
  Vec/1 -> Dot Product/2, Dot Product/1
